simulink model "SzSolo_ultimo"  (R2021b)
settings: Solver=VariableStepAuto  StartTime=0.0  StopTime=1  RelTol=1e-3
PreLoadFcn:
  | Fs = 44100;
  | L = 32;
InitFcn:
  | Fs = 44100;
  | L = 32;
StopFcn:
  | size_ws = size(out.ws);
  | n_rows = size_ws(1);
  | SzEstimado = out.ws(n_rows, :);
libraries: dspsrcs4 x1
settings Model: Creator=Vale Oieni  LastModifiedBy=ValeOieni

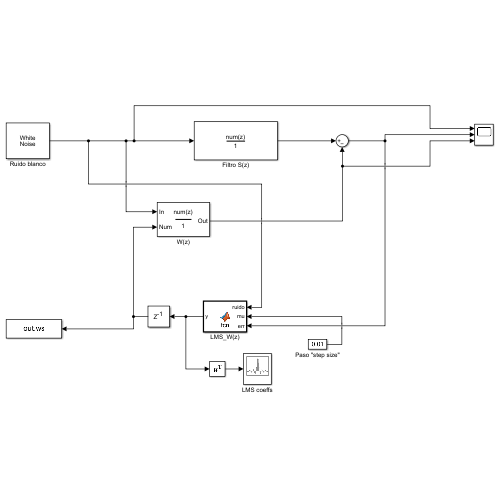
[thumbnail: Simulink's stored preview of the top-level diagram]
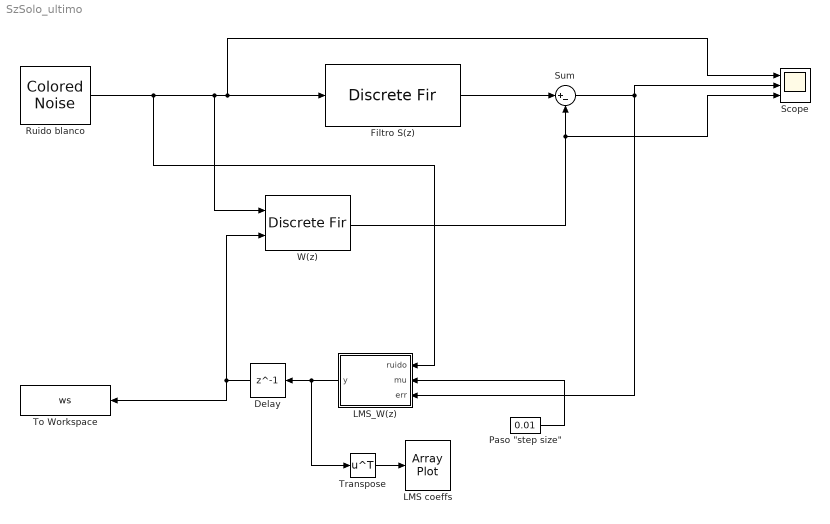
== system SzSolo_ultimo ==
  Delay : Delay  DelayLength=1  InitialCondition=0
  Filtro S(z) : DiscreteFir  Coefficients=[0 0 -.5 .5 -.3 .2 -.1 .5 -.5]  InputProcessing=Columns as channels (frame based)  SampleTime=1/Fs
  LMS coeffs : ArrayPlot  WindowPosition=[794.000000,30.000000,798.000000,828.000000,]  Visible=on  AxesScaling=Manual  YLimits=[-0.624999,0.624999]  ShowLegend=on  DefaultConfigurationName=dsp.scopes.ArrayPlotBlockSpecification
  LMS_W(z) : MATLAB Function  TreatAsAtomicUnit=on
  "Paso \"step size\"" : Constant  Value=0.01  SampleTime=1/Fs
  Ruido blanco : dspsrcs4/Colored Noise  Color=white  InverseFrequencyPower=1  BoundedOutput=off  NumChannels=1  OutputDataType=double  SamplesPerFrame=1  SampleTime=1/Fs  RandomStream=mt19937ar with seed  Seed=67  SimulateUsing=Interpreted execution
      settings: SourceProductBaseCode=DS
  Scope : Scope  NumInputPorts=3
  Sum : Sum  Inputs=|+-
  To Workspace : ToWorkspace  VariableName=ws  SampleTime=-1
      settings: Save2DSignal=2-D array (concatenate along first dimension)
  Transpose : Math  Operator=transpose  SignedPower=on  SaturateOnIntegerOverflow=on
  W(z) : DiscreteFir  CoefSource=Input port  SampleTime=1/Fs
      settings: InputPortMap=u0,u1
  wires:
  Ruido blanco/1 -> W(z)/1, Scope/1, Filtro S(z)/1, LMS_W(z)/1(ruido)
  Sum/1 -> LMS_W(z)/3(err), Scope/2
  Filtro S(z)/1 -> Sum/1
  W(z)/1 -> Scope/3, Sum/2
  Delay/1 -> W(z)/2, To Workspace/1
  LMS_W(z)/1(y) -> Transpose/1, Delay/1
  Transpose/1 -> LMS coeffs/1
  "Paso \"step size\""/1 -> LMS_W(z)/2(mu)

== matlab function SzSolo_ultimo/LMS_W(z) ==
  data: ruido input; mu input; y output; err input
function y = fcn(ruido, mu, err)
    L = 32;
    %Pesos w_n
    persistent w_n
    if isempty(w_n)
        w_n = zeros(1, L); % inicializa w en cero, largo L
    end
    %Vector de ruido
    persistent x
    if isempty(x)
        x = zeros(1, L); % inicializa x en cero, largo L
    end
    %Vaciado de x
    x(2:L) = x(1:L-1);
    x(1) = ruido;
    %Actualizacion
    xvar = x;
    w = w_n;
    w = w + mu*err*xvar;   
    w_n = w;
    %Asignación a la salida
    y = w;
end
